simulink model "bpsk"  (R2018b)
settings: Solver=VariableStepAuto  StartTime=0.0  StopTime=0  RelTol=1e-3
libraries: commrandsrc3 x1
settings Model: Creator=DSP_27  LastModifiedBy=DSP_27

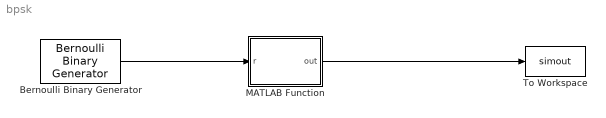
== system bpsk ==
  Bernoulli Binary Generator : commrandsrc3/Bernoulli Binary Generator  ProbabilityOfZero=0.5  SeedSource=Auto  Seed=0  SampleTime=1  SamplesPerFrame=1000  OutputDataType=double  SimulateUsing=Interpreted execution
  MATLAB Function : MATLAB Function  TreatAsAtomicUnit=on
  To Workspace : ToWorkspace  VariableName=simout  SampleTime=-1
      settings: Save2DSignal=2-D array (concatenate along first dimension)
  wires:
  Bernoulli Binary Generator/1 -> MATLAB Function/1(r)
  MATLAB Function/1(out) -> To Workspace/1

== matlab function bpsk/MATLAB Function ==
  data: r input; out output
function out = fcn(r)


N = length(r);

%N=10000;
z= zeros(length(r),1);

y =zeros(1, length(r));
%r = randi([0,1],N,1);

for i=1:N                     %converted to bpsk
    
        if(r(i)==0) 
            r(i) = -1;
        else
             r(i) = 1;
        end
    

end

n = randn(N,1);                 %noise signal


snr_db = 0:2:24;     
kk=1;% snr in db

ber_prac = zeros(1, length(snr_db));

for k = 1: length(snr_db)
    
snr_linear = 10.^(snr_db(k)/10);           % converted snr to linear
sigma = 1./(snr_linear).^(1/2);                % find sigma

y = r+ sigma.*n;                 % find y = bpsk_signal + sigma*noise


% convert y sequence into bpsk take threshold value = 0
% z is your constructed signal
% y is output signal with noise
for j=1:N
   if(y(j)<0) 
            z(j,1) = -1;
        else
            z(j,1) = 1;
        end

end

% check bit by bit that r and z is same or not

count_error=0;
for jj=1:N
    if(r(jj)~=z(jj))
        count_error=count_error+1;
%     else
%         count_error;
    end
end

% calculate theortical ber  Q((snr_linear)^(1/2)


%ber_th(k) = qfunc((snr_linear).^(1/2));
ber_prac(k) = count_error/N;
%k=k+1;
end



out = ber_prac;
